simulink model "Guidance"  (Simulink 8.8)
settings: Solver=ode4  StartTime=0.0  StopTime=100  FixedStep=0.001  RelTol=1e-3
values from neighbouring files (symbols this model uses):
  direction_vm = -180 * Deg2Rad    (= -3.14159265359)    [Initialize.m]
  direction_vt = 0    [Initialize.m]
  K_Guide = 3    [Initialize.m]
  latex_t = 2    [Initialize.m]
  Vm = 850    [Initialize.m]
  Vt = 300    [Initialize.m]
  xm0 = 30000    [Initialize.m]
  xt0 = 0    [Initialize.m]
  ym0 = 5000    [Initialize.m]
  yt0 = 0    [Initialize.m]
undefined symbols (not defined in the file or in its folder): Vmx0, Vmy0
libraries: simulink x1
settings Model: Creator=SH  LastModifiedBy=SH
settings DataIOCC: LimitDataPoints=off  SaveFormat=Dataset  SignalLoggingSaveFormat=Dataset
settings OptimizationCC: LifeSpan=auto
settings DebuggingCC: UnderspecifiedInitializationDetection=Simplified  MergeDetectMultiDrivingBlocksExec=error  FcnCallInpInsideContextMsg=error  StateNameClashWarn=none  SFUnexpectedBacktrackingDiag=error  SFNoUnconditionalDefaultTransitionDiag=error  SFExecutionAtInitializationDiag=warning
settings HardwareCC: ProdBitPerPointer=64  ProdBitPerSizeT=64  ProdBitPerPtrDiffT=64  ProdLargestAtomicFloat=Float  ProdIntDivRoundTo=Zero  ProdEndianess=LittleEndian  ProdWordSize=64  ProdHWDeviceType=Intel->x86-64 (Windows64)
settings ModelReferenceCC: PropagateSignalLabelsOutOfModel=on
settings GRTTargetCC: TargetLangStandard=C99 (ISO)  GeneratePreprocessorConditionals=Use local settings  CombineOutputUpdateFcns=on  GRTInterface=off
settings ConfigComp: CovMetricSettings=dwe  CovHtmlReporting=off  CovSaveCumulativeToWorkspaceVar=off  CovSaveSingleToWorkspaceVar=off  CovExternalEMLEnable=on

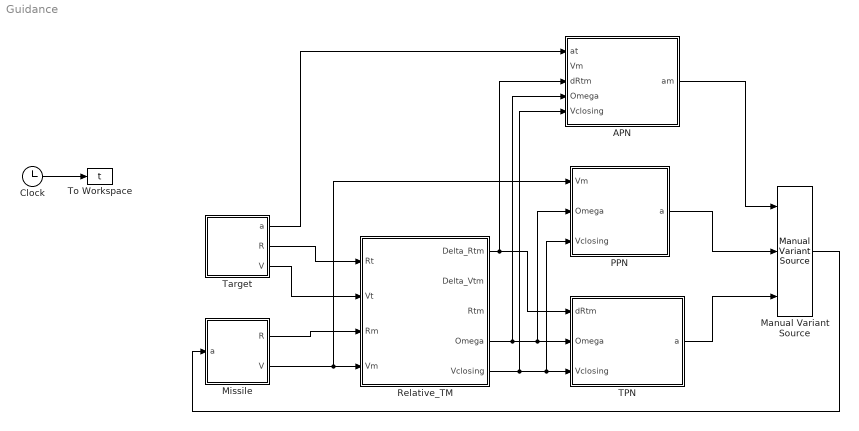
== system Guidance ==
  APN : Subsystem
  Clock : Clock
  Manual Variant Source : simulink/Signal Routing/Manual Variant Source  NumChoices=3  OverrideUsingVariant=V_1
  Missile : Subsystem
  PPN : Subsystem
  Relative_TM : Subsystem
  TPN : Subsystem
  Target : Subsystem
  To Workspace : ToWorkspace  VariableName=t  SampleTime=-1
  wires:
  Target/2(R) -> Relative_TM/1(Rt)
  Target/3(V) -> Relative_TM/2(Vt)
  Missile/1(R) -> Relative_TM/3(Rm)
  Missile/2(V) -> PPN/1(Vm), Relative_TM/4(Vm)
  Relative_TM/1(Delta_Rtm) -> APN/3(dRtm), TPN/1(dRtm)
  Relative_TM/4(Omega) -> APN/4(Omega), PPN/2(Omega), TPN/2(Omega)
  Relative_TM/5(Vclosing) -> APN/5(Vclosing), PPN/3(Vclosing), TPN/3(Vclosing)
  Manual Variant Source/1 -> Missile/1(a)
  Clock/1 -> To Workspace/1
  PPN/1(a) -> Manual Variant Source/2
  TPN/1(a) -> Manual Variant Source/3
  APN/1(am) -> Manual Variant Source/1
  Target/1(a) -> APN/1(at)

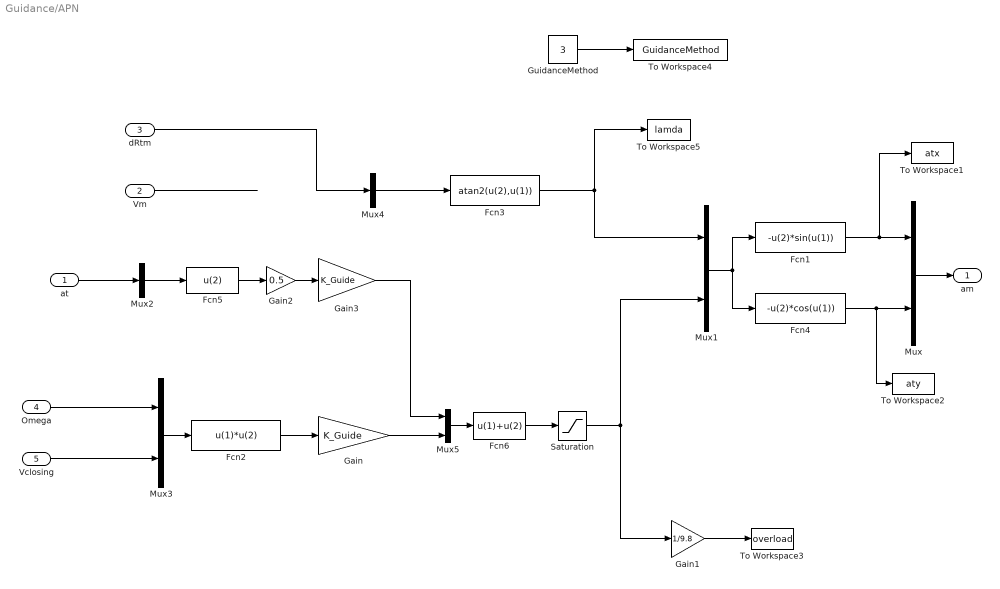
== system Guidance/APN ==
  at : Inport
  Vm : Inport  Port=2
  dRtm : Inport  Port=3
  Omega : Inport  Port=4
  Vclosing : Inport  Port=5
  Fcn1 : Fcn  Expr=-u(2)*sin(u(1))
  Fcn2 : Fcn  Expr=u(1)*u(2)
  Fcn3 : Fcn  Expr=atan2(u(2),u(1))
  Fcn4 : Fcn  Expr=-u(2)*cos(u(1))
  Fcn5 : Fcn  Expr=u(2)
  Fcn6 : Fcn  Expr=u(1)+u(2)
  Gain : Gain  Gain=K_Guide
  Gain1 : Gain  Gain=1/9.8
  Gain2 : Gain  Gain=0.5
  Gain3 : Gain  Gain=K_Guide
  GuidanceMethod : Constant  Value=3
  Mux{,1,3,5} (4 alike) : Mux  Inputs=2
  Mux2 : Mux  Inputs=1
  Mux4 : Mux  Inputs=1
  Saturation : Saturate  UpperLimit=40*9.8  LowerLimit=-40*9.8
  To Workspace1 : ToWorkspace  VariableName=atx  SampleTime=-1
  To Workspace2 : ToWorkspace  VariableName=aty  SampleTime=-1
  To Workspace3 : ToWorkspace  VariableName=overload  SampleTime=-1
  To Workspace4 : ToWorkspace  VariableName=GuidanceMethod  SampleTime=-1
  To Workspace5 : ToWorkspace  VariableName=lamda  SampleTime=-1
  am : Outport
  wires:
  Saturation/1 -> Mux1/2, Gain1/1
  Fcn4/1 -> Mux/2, To Workspace2/1
  Fcn1/1 -> Mux/1, To Workspace1/1
  Mux1/1 -> Fcn1/1, Fcn4/1
  Mux/1 -> am/1
  Fcn3/1 -> To Workspace5/1, Mux1/1
  Mux4/1 -> Fcn3/1
  dRtm/1 -> Mux4/1
  Gain1/1 -> To Workspace3/1
  Gain/1 -> Mux5/2
  Mux3/1 -> Fcn2/1
  Fcn2/1 -> Gain/1
  Vclosing/1 -> Mux3/2
  Omega/1 -> Mux3/1
  Mux2/1 -> Fcn5/1
  at/1 -> Mux2/1
  Fcn5/1 -> Gain2/1
  Gain2/1 -> Gain3/1
  Gain3/1 -> Mux5/1
  Mux5/1 -> Fcn6/1
  Fcn6/1 -> Saturation/1
  GuidanceMethod/1 -> To Workspace4/1
  Vm/1 -> ?

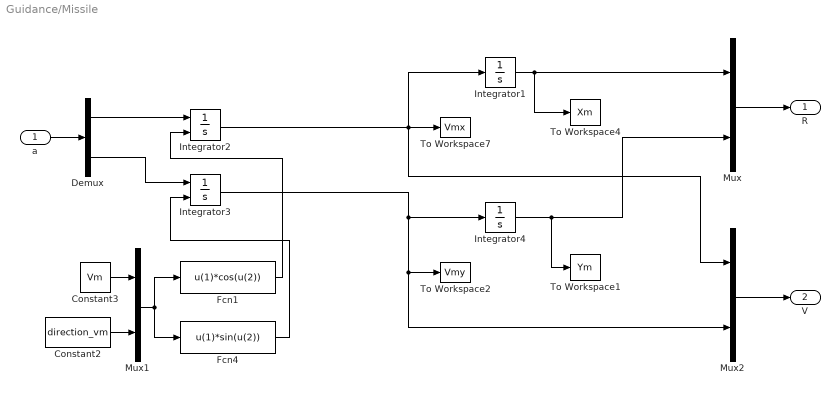
== system Guidance/Missile ==
  a : Inport
  Constant2 : Constant  Value=direction_vm
  Constant3 : Constant  Value=Vm
  Demux : Demux  Outputs=2
  Fcn1 : Fcn  Expr=u(1)*cos(u(2))
  Fcn4 : Fcn  Expr=u(1)*sin(u(2))
  Integrator1 : Integrator  InitialCondition=xm0
  Integrator2 : Integrator  InitialConditionSource=external  InitialCondition=Vmx0
  Integrator3 : Integrator  InitialConditionSource=external  InitialCondition=Vmy0
  Integrator4 : Integrator  InitialCondition=ym0
  Mux : Mux  Inputs=2
  Mux1 : Mux  Inputs=2
  Mux2 : Mux  Inputs=2
  To Workspace1 : ToWorkspace  VariableName=Ym  SampleTime=-1
  To Workspace2 : ToWorkspace  VariableName=Vmy  SampleTime=-1
  To Workspace4 : ToWorkspace  VariableName=Xm  SampleTime=-1
  To Workspace7 : ToWorkspace  VariableName=Vmx  SampleTime=-1
  R : Outport
  V : Outport  Port=2
  wires:
  Mux/1 -> R/1
  Integrator1/1 -> Mux/1, To Workspace4/1
  Integrator4/1 -> Mux/2, To Workspace1/1
  Integrator3/1 -> Integrator4/1, Mux2/2, To Workspace2/1
  Mux1/1 -> Fcn4/1, Fcn1/1
  Integrator2/1 -> Integrator1/1, Mux2/1, To Workspace7/1
  Constant2/1 -> Mux1/2
  Constant3/1 -> Mux1/1
  Mux2/1 -> V/1
  Fcn1/1 -> Integrator2/2
  a/1 -> Demux/1
  Demux/1 -> Integrator2/1
  Demux/2 -> Integrator3/1
  Fcn4/1 -> Integrator3/2

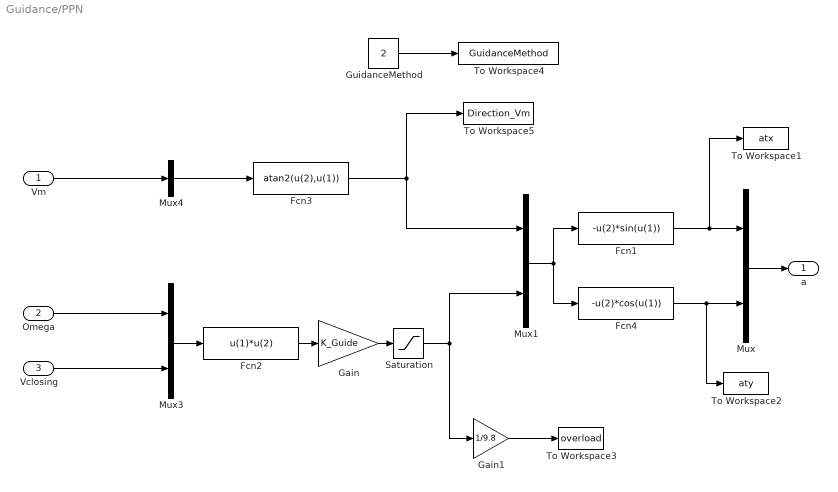
== system Guidance/PPN ==
  Vm : Inport
  Omega : Inport  Port=2
  Vclosing : Inport  Port=3
  Fcn1 : Fcn  Expr=-u(2)*sin(u(1))
  Fcn2 : Fcn  Expr=u(1)*u(2)
  Fcn3 : Fcn  Expr=atan2(u(2),u(1))
  Fcn4 : Fcn  Expr=-u(2)*cos(u(1))
  Gain : Gain  Gain=K_Guide
  Gain1 : Gain  Gain=1/9.8
  GuidanceMethod : Constant  Value=2
  Mux : Mux  Inputs=2
  Mux1 : Mux  Inputs=2
  Mux3 : Mux  Inputs=2
  Mux4 : Mux  Inputs=1
  Saturation : Saturate  UpperLimit=40*9.8  LowerLimit=-40*9.8
  To Workspace1 : ToWorkspace  VariableName=atx  SampleTime=-1
  To Workspace2 : ToWorkspace  VariableName=aty  SampleTime=-1
  To Workspace3 : ToWorkspace  VariableName=overload  SampleTime=-1
  To Workspace4 : ToWorkspace  VariableName=GuidanceMethod  SampleTime=-1
  To Workspace5 : ToWorkspace  VariableName=Direction_Vm  SampleTime=-1
  a : Outport
  wires:
  Omega/1 -> Mux3/1
  Vclosing/1 -> Mux3/2
  Fcn2/1 -> Gain/1
  Mux3/1 -> Fcn2/1
  Gain/1 -> Saturation/1
  Gain1/1 -> To Workspace3/1
  Vm/1 -> Mux4/1
  Mux4/1 -> Fcn3/1
  Fcn3/1 -> Mux1/1, To Workspace5/1
  Mux/1 -> a/1
  Mux1/1 -> Fcn4/1, Fcn1/1
  Fcn1/1 -> To Workspace1/1, Mux/1
  Fcn4/1 -> To Workspace2/1, Mux/2
  Saturation/1 -> Mux1/2, Gain1/1
  GuidanceMethod/1 -> To Workspace4/1

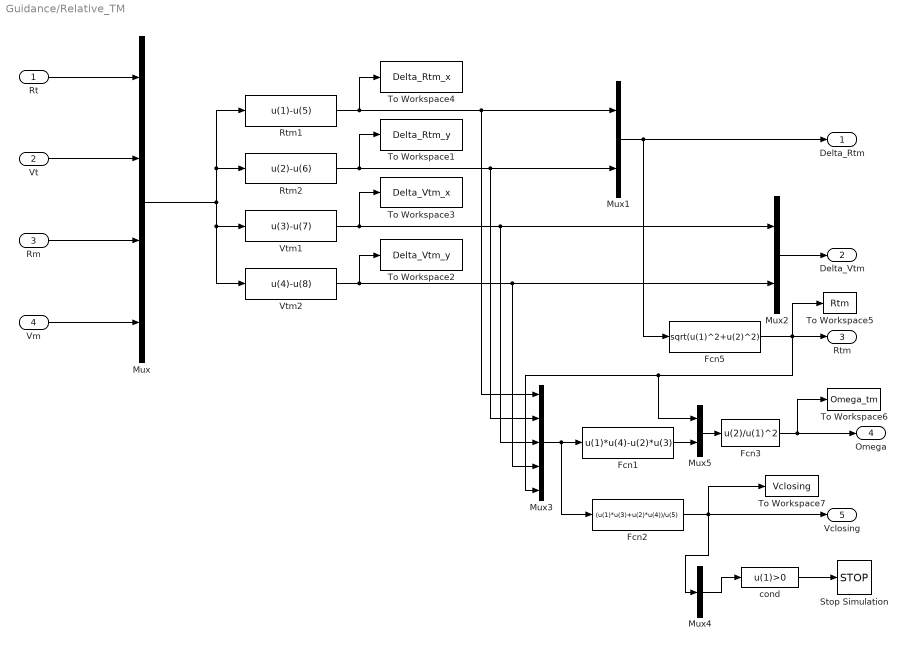
== system Guidance/Relative_TM ==
  Rt : Inport
  Vt : Inport  Port=2
  Rm : Inport  Port=3
  Vm : Inport  Port=4
  Fcn1 : Fcn  Expr=u(1)*u(4)-u(2)*u(3)
  Fcn2 : Fcn  Expr=(u(1)*u(3)+u(2)*u(4))/u(5)
  Fcn3 : Fcn  Expr=u(2)/u(1)^2
  Fcn5 : Fcn  Expr=sqrt(u(1)^2+u(2)^2)
  Mux : Mux
  Mux1 : Mux  Inputs=2
  Mux2 : Mux  Inputs=2
  Mux3 : Mux  Inputs=5
  Mux4 : Mux  Inputs=1
  Mux5 : Mux  Inputs=2
  Rtm1 : Fcn  Expr=u(1)-u(5)
  Rtm2 : Fcn  Expr=u(2)-u(6)
  Stop Simulation : Stop
  To Workspace1 : ToWorkspace  VariableName=Delta_Rtm_y  SampleTime=-1
  To Workspace2 : ToWorkspace  VariableName=Delta_Vtm_y  SampleTime=-1
  To Workspace3 : ToWorkspace  VariableName=Delta_Vtm_x  SampleTime=-1
  To Workspace4 : ToWorkspace  VariableName=Delta_Rtm_x  SampleTime=-1
  To Workspace5 : ToWorkspace  VariableName=Rtm  SampleTime=-1
  To Workspace6 : ToWorkspace  VariableName=Omega_tm  SampleTime=-1
  To Workspace7 : ToWorkspace  VariableName=Vclosing  SampleTime=-1
  Vtm1 : Fcn  Expr=u(3)-u(7)
  Vtm2 : Fcn  Expr=u(4)-u(8)
  cond : Fcn  Expr=u(1)>0
  Delta_Rtm : Outport
  Delta_Vtm : Outport  Port=2
  Rtm : Outport  Port=3
  Omega : Outport  Port=4
  Vclosing : Outport  Port=5
  wires:
  Vm/1 -> Mux/4
  Rm/1 -> Mux/3
  Vt/1 -> Mux/2
  Rt/1 -> Mux/1
  Mux/1 -> Vtm2/1, Vtm1/1, Rtm1/1, Rtm2/1
  Rtm1/1 -> Mux3/1, Mux1/1, To Workspace4/1
  Rtm2/1 -> Mux3/2, Mux1/2, To Workspace1/1
  Vtm1/1 -> Mux3/3, Mux2/1, To Workspace3/1
  Vtm2/1 -> Mux3/4, Mux2/2, To Workspace2/1
  Mux1/1 -> Fcn5/1, Delta_Rtm/1
  Mux2/1 -> Delta_Vtm/1
  Fcn5/1 -> Mux5/1, Mux3/5, To Workspace5/1, Rtm/1
  Mux3/1 -> Fcn2/1, Fcn1/1
  Fcn1/1 -> Mux5/2
  Fcn2/1 -> Mux4/1, To Workspace7/1, Vclosing/1
  cond/1 -> Stop Simulation/1
  Mux4/1 -> cond/1
  Fcn3/1 -> To Workspace6/1, Omega/1
  Mux5/1 -> Fcn3/1

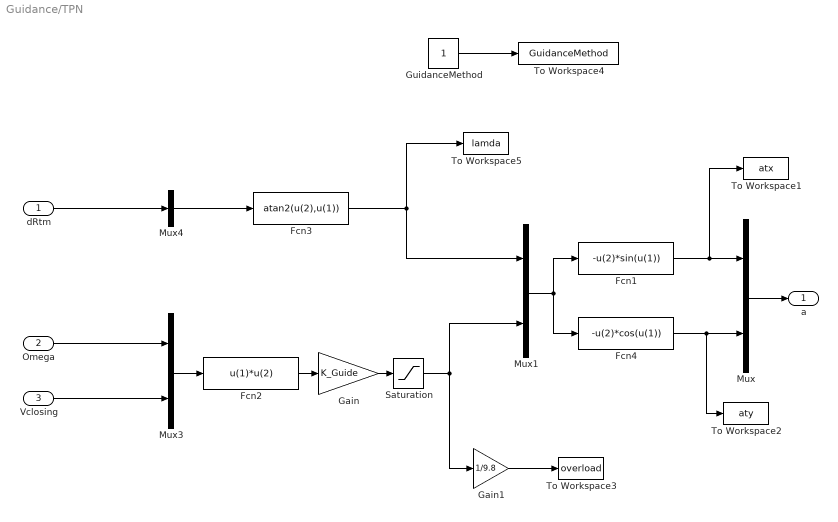
== system Guidance/TPN ==
  dRtm : Inport
  Omega : Inport  Port=2
  Vclosing : Inport  Port=3
  Fcn1 : Fcn  Expr=-u(2)*sin(u(1))
  Fcn2 : Fcn  Expr=u(1)*u(2)
  Fcn3 : Fcn  Expr=atan2(u(2),u(1))
  Fcn4 : Fcn  Expr=-u(2)*cos(u(1))
  Gain : Gain  Gain=K_Guide
  Gain1 : Gain  Gain=1/9.8
  GuidanceMethod : Constant
  Mux : Mux  Inputs=2
  Mux1 : Mux  Inputs=2
  Mux3 : Mux  Inputs=2
  Mux4 : Mux  Inputs=1
  Saturation : Saturate  UpperLimit=40*9.8  LowerLimit=-40*9.8
  To Workspace1 : ToWorkspace  VariableName=atx  SampleTime=-1
  To Workspace2 : ToWorkspace  VariableName=aty  SampleTime=-1
  To Workspace3 : ToWorkspace  VariableName=overload  SampleTime=-1
  To Workspace4 : ToWorkspace  VariableName=GuidanceMethod  SampleTime=-1
  To Workspace5 : ToWorkspace  VariableName=lamda  SampleTime=-1
  a : Outport
  wires:
  Omega/1 -> Mux3/1
  Vclosing/1 -> Mux3/2
  Fcn2/1 -> Gain/1
  Mux3/1 -> Fcn2/1
  Gain/1 -> Saturation/1
  Gain1/1 -> To Workspace3/1
  dRtm/1 -> Mux4/1
  Mux4/1 -> Fcn3/1
  Fcn3/1 -> Mux1/1, To Workspace5/1
  Mux/1 -> a/1
  Mux1/1 -> Fcn4/1, Fcn1/1
  Fcn1/1 -> To Workspace1/1, Mux/1
  Fcn4/1 -> To Workspace2/1, Mux/2
  Saturation/1 -> Mux1/2, Gain1/1
  GuidanceMethod/1 -> To Workspace4/1

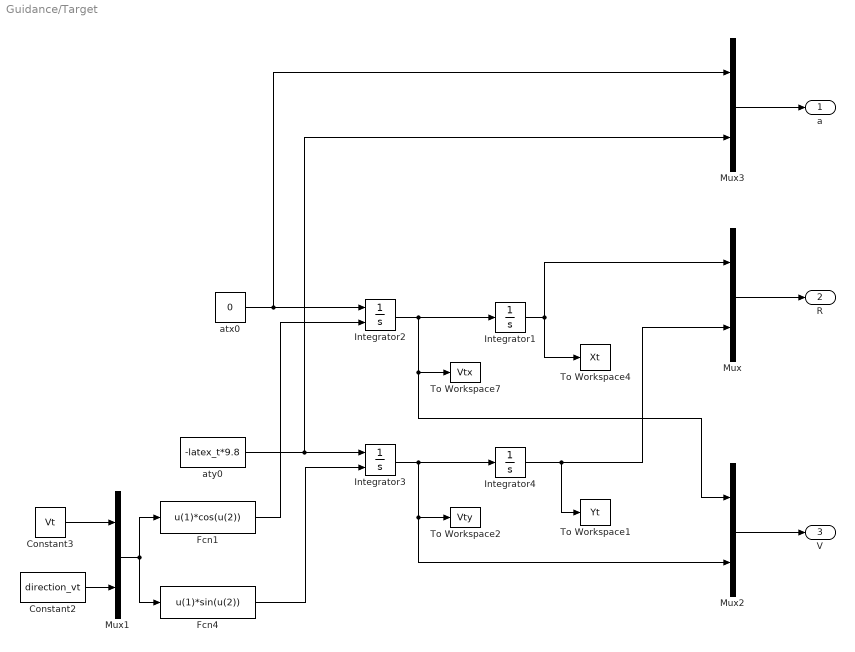
== system Guidance/Target ==
  Constant2 : Constant  Value=direction_vt
  Constant3 : Constant  Value=Vt
  Fcn1 : Fcn  Expr=u(1)*cos(u(2))
  Fcn4 : Fcn  Expr=u(1)*sin(u(2))
  Integrator1 : Integrator  InitialCondition=xt0
  Integrator2 : Integrator  InitialConditionSource=external  InitialCondition=xt0
  Integrator3 : Integrator  InitialConditionSource=external  InitialCondition=xt0
  Integrator4 : Integrator  InitialCondition=yt0
  Mux{,1..3} (4 alike) : Mux  Inputs=2
  To Workspace1 : ToWorkspace  VariableName=Yt  SampleTime=-1
  To Workspace2 : ToWorkspace  VariableName=Vty  SampleTime=-1
  To Workspace4 : ToWorkspace  VariableName=Xt  SampleTime=-1
  To Workspace7 : ToWorkspace  VariableName=Vtx  SampleTime=-1
  atx0 : Constant  Value=0
  aty0 : Constant  Value=-latex_t*9.8
  a : Outport
  R : Outport  Port=2
  V : Outport  Port=3
  wires:
  Constant3/1 -> Mux1/1
  Constant2/1 -> Mux1/2
  Integrator2/1 -> Mux2/1, To Workspace7/1, Integrator1/1
  Mux1/1 -> Fcn4/1, Fcn1/1
  Integrator3/1 -> Mux2/2, To Workspace2/1, Integrator4/1
  Integrator4/1 -> To Workspace1/1, Mux/2
  Integrator1/1 -> To Workspace4/1, Mux/1
  Mux/1 -> R/1
  Mux2/1 -> V/1
  aty0/1 -> Mux3/2, Integrator3/1
  atx0/1 -> Mux3/1, Integrator2/1
  Fcn1/1 -> Integrator2/2
  Fcn4/1 -> Integrator3/2
  Mux3/1 -> a/1
